simulink model "IPG"  (R2019a)
settings: Solver=FixedStepDiscrete  StartTime=0.0  StopTime=86.24  FixedStep=0.01  RelTol=1e-3
undefined symbols (not defined in the file): C1Prime, C2Prime, C3Prime, CapacityAh, DiscIntNeverNeededParam, Em, InitialCapVoltage, R0, Rx, SOC_LUT
settings Model: Creator=danis  LastModifiedBy=danis

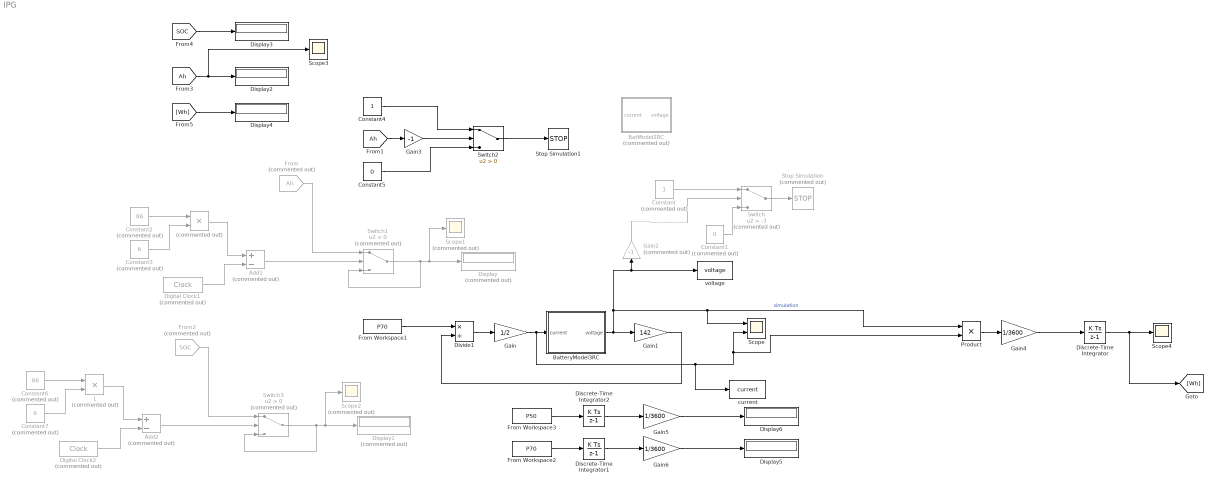
== system IPG ==
  " " : Product  Commented=on  Inputs=**
  " 1" : Product  Commented=on  Inputs=**
  Add1 : Sum  Commented=on  Inputs=+-
  Add2 : Sum  Commented=on  Inputs=+-
  BatModel2RC : Subsystem  Commented=on
  BatteryModel3RC : Subsystem
  Constant : Constant  Commented=on  SampleTime=0.01
  Constant1 : Constant  Commented=on  Value=0  SampleTime=0.01
  Constant2 : Constant  Commented=on  Value=86  SampleTime=0.01
  Constant3 : Constant  Commented=on  Value=6  SampleTime=0.01
  Constant4 : Constant  SampleTime=0.01
  Constant5 : Constant  Value=0  SampleTime=0.01
  Constant6 : Constant  Commented=on  Value=86  SampleTime=0.01
  Constant7 : Constant  Commented=on  Value=6  SampleTime=0.01
  Digital Clock1 : DigitalClock  Commented=on  SampleTime=0.01
  Digital Clock2 : DigitalClock  Commented=on  SampleTime=0.01
  Discrete-Time Integrator : DiscreteIntegrator  SampleTime=-1  ICPrevOutput=DiscIntNeverNeededParam  ICPrevScaledInput=DiscIntNeverNeededParam
  Discrete-Time Integrator1 : DiscreteIntegrator  SampleTime=-1  ICPrevOutput=DiscIntNeverNeededParam  ICPrevScaledInput=DiscIntNeverNeededParam
  Discrete-Time Integrator2 : DiscreteIntegrator  SampleTime=-1  ICPrevOutput=DiscIntNeverNeededParam  ICPrevScaledInput=DiscIntNeverNeededParam
  Display : Display  Commented=on
  Display1 : Display  Commented=on
  Display{2..6} (5 alike) : Display
  Divide1 : Product  Inputs=*/
  From : From  Commented=on  GotoTag=Ah  TagVisibility=global
  From Workspace1 : FromWorkspace  VariableName=P70  SampleTime=0.01  Interpolate=off  OutputAfterFinalValue=Cyclic repetition
  From Workspace2 : FromWorkspace  VariableName=P70  SampleTime=0.01  Interpolate=off  OutputAfterFinalValue=Cyclic repetition
  From Workspace3 : FromWorkspace  VariableName=P50  SampleTime=0.01  Interpolate=off  OutputAfterFinalValue=Cyclic repetition
  From2 : From  Commented=on  GotoTag=SOC  TagVisibility=global
  Gain : Gain  Gain=1/2
  Gain1 : Gain  Gain=142
  Gain2 : Gain  Commented=on  Gain=-1
  Gain3 : Gain  Gain=-1
  Gain4 : Gain  Gain=1/3600
  Gain5 : Gain  Gain=1/3600
  Gain6 : Gain  Gain=1/3600
  Product : Product
  Scope : Scope  NumInputPorts=2
  Scope1 : Scope  Commented=on
  Scope2 : Scope  Commented=on
  Scope3 : Scope
  Scope4 : Scope
  Stop Simulation : Stop  Commented=on
  Stop Simulation1 : Stop
  Switch : Switch  Commented=on  Criteria=u2 > Threshold  Threshold=-3
  Switch1 : Switch  Commented=on  Criteria=u2 > Threshold
  Switch2 : Switch  Criteria=u2 > Threshold
  Switch3 : Switch  Commented=on  Criteria=u2 > Threshold
  current : ToWorkspace  VariableName=current  SaveFormat=Structure With Time  SampleTime=-1
  voltage : ToWorkspace  VariableName=voltage  SaveFormat=Structure With Time  SampleTime=-1
  wires:
  Divide1/1 -> Gain/1
  Gain/1 -> BatteryModel3RC/1(current), current/1, Scope/2, Product/2
  Gain1/1 -> Divide1/2
  Switch/1 -> Stop Simulation/1
  Gain2/1 -> Switch/2
  Constant/1 -> Switch/1
  Constant1/1 -> Switch/3
  From Workspace1/1 -> Divide1/1
  From/1 -> Switch1/1
  Add1/1 -> Switch1/2
  Switch1/1 -> Switch1/3, Scope1/1, Display/1
  Constant2/1 -> " "/1
  Constant3/1 -> " "/2
  " "/1 -> Add1/1
  Digital Clock1/1 -> Add1/2
  [Ah] -> Gain3/1
  Constant4/1 -> Switch2/1
  Constant5/1 -> Switch2/3
  Switch2/1 -> Stop Simulation1/1
  Digital Clock2/1 -> Add2/2
  " 1"/1 -> Add2/1
  Constant7/1 -> " 1"/2
  Constant6/1 -> " 1"/1
  Switch3/1 -> Display1/1, Scope2/1, Switch3/3
  Add2/1 -> Switch3/2
  From2/1 -> Switch3/1
  Gain3/1 -> Switch2/2
  [Ah] -> Scope3/1, Display2/1
  [SOC] -> Display3/1
  Discrete-Time Integrator/1 -> [Wh], Scope4/1
  Gain4/1 -> Discrete-Time Integrator/1
  Product/1 -> Gain4/1
  [Wh] -> Display4/1
  BatteryModel3RC/1(voltage) -> Gain1/1, Product/1, Scope/1, voltage/1, Gain2/1  "simulation"
  From Workspace2/1 -> Discrete-Time Integrator1/1
  Discrete-Time Integrator1/1 -> Gain6/1
  Gain6/1 -> Display5/1
  Gain5/1 -> Display6/1
  Discrete-Time Integrator2/1 -> Gain5/1
  From Workspace3/1 -> Discrete-Time Integrator2/1

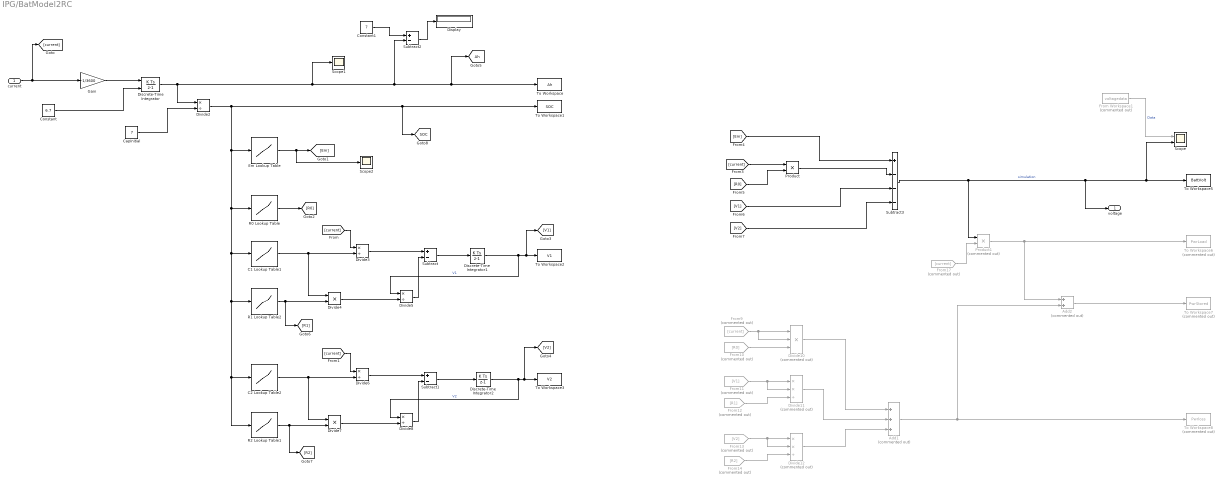
== system IPG/BatModel2RC ==
  current : Inport
  Add1 : Sum  Commented=on  Inputs=+++
  Add2 : Sum  Commented=on
  C1 Lookup Table1 : Lookup_n-D  NumberOfTableDimensions=1  BreakpointsForDimension1=SOC_LUT  Table=C1Prime(1,:)  InternalRulePriority=Speed  RndMeth=Simplest  InputSameDT=on
  C2 Lookup Table2 : Lookup_n-D  NumberOfTableDimensions=1  BreakpointsForDimension1=SOC_LUT  Table=C2Prime(1,:)  InternalRulePriority=Speed  RndMeth=Simplest  InputSameDT=on
  CapInitial : Constant  Value=7  SampleTime=-1
  Constant : Constant  Value=6.7  SampleTime=-1
  Constant1 : Constant  Value=7  SampleTime=0.01
  Discrete-Time Integrator : DiscreteIntegrator  InitialConditionSource=external  SampleTime=-1  ICPrevOutput=DiscIntNeverNeededParam  ICPrevScaledInput=DiscIntNeverNeededParam
  Discrete-Time Integrator1 : DiscreteIntegrator  InitialCondition=InitialCapVoltage(1)  SampleTime=-1  ICPrevOutput=DiscIntNeverNeededParam  ICPrevScaledInput=DiscIntNeverNeededParam
  Discrete-Time Integrator2 : DiscreteIntegrator  InitialCondition=InitialCapVoltage(2)  SampleTime=-1  ICPrevOutput=DiscIntNeverNeededParam  ICPrevScaledInput=DiscIntNeverNeededParam
  Display : Display
  Divide10 : Product  Commented=on  Inputs=***
  Divide11 : Product  Commented=on  Inputs=**/
  Divide12 : Product  Commented=on  Inputs=**/
  Divide{2..3,5..6,8} (5 alike) : Product  Inputs=*/
  Divide4 : Product  Inputs=**
  Divide7 : Product  Inputs=**
  Em Lookup Table : Lookup_n-D  NumberOfTableDimensions=1  BreakpointsForDimension1=SOC_LUT  Table=Em  InternalRulePriority=Speed  RndMeth=Simplest  InputSameDT=on
  From Workspace1 : FromWorkspace  Commented=on  VariableName=voltagedata  SampleTime=0.001
  From10 : From  Commented=on  GotoTag=R0
  From11 : From  Commented=on  GotoTag=V1
  From12 : From  Commented=on  GotoTag=R1
  From13 : From  Commented=on  GotoTag=V2
  From14 : From  Commented=on  GotoTag=R2
  From17 : From  Commented=on  GotoTag=current
  From9 : From  Commented=on  GotoTag=current
  Gain : Gain  Gain=-1/3600
  Product : Product
  Product1 : Product  Commented=on
  R0 Lookup Table : Lookup_n-D  NumberOfTableDimensions=1  BreakpointsForDimension1=SOC_LUT  Table=R0  InternalRulePriority=Speed  RndMeth=Simplest  InputSameDT=on
  R1 Lookup Table2 : Lookup_n-D  NumberOfTableDimensions=1  BreakpointsForDimension1=SOC_LUT  Table=Rx(1,:)  InternalRulePriority=Speed  RndMeth=Simplest  InputSameDT=on
  R2 Lookup Table1 : Lookup_n-D  NumberOfTableDimensions=1  BreakpointsForDimension1=SOC_LUT  Table=Rx(2,:)  InternalRulePriority=Speed  RndMeth=Simplest  InputSameDT=on
  Scope : Scope  NumInputPorts=2
  Scope1 : Scope
  Scope2 : Scope
  Subtract : Sum  Inputs=+-
  Subtract1 : Sum  Inputs=+-
  Subtract2 : Sum  Inputs=+-
  Subtract3 : Sum  Inputs=+---
  To Workspace : ToWorkspace  VariableName=Ah  SampleTime=-1
  To Workspace1 : ToWorkspace  VariableName=SOC  SampleTime=-1
  To Workspace2 : ToWorkspace  VariableName=V1  SampleTime=-1
  To Workspace3 : ToWorkspace  VariableName=V2  SampleTime=-1
  To Workspace5 : ToWorkspace  VariableName=BattVolt  SampleTime=-1
  To Workspace6 : ToWorkspace  Commented=on  VariableName=PwrLoad  SampleTime=-1
  To Workspace7 : ToWorkspace  Commented=on  VariableName=PwrStored  SampleTime=-1
  To Workspace8 : ToWorkspace  Commented=on  VariableName=Pwrloss  SampleTime=-1
  voltage : Outport
  tag scope: Ah=global, SOC=global
  wires:
  Gain/1 -> Discrete-Time Integrator/1
  Discrete-Time Integrator/1 -> Scope1/1, Subtract2/2, [Ah], To Workspace/1, Divide2/1
  Divide10/1 -> Add1/1
  Discrete-Time Integrator1/1 -> Divide5/1, To Workspace2/1, [V1]  "V1"
  Divide2/1 -> [SOC], To Workspace1/1, R2 Lookup Table1/1, C2 Lookup Table2/1, R1 Lookup Table2/1, C1 Lookup Table1/1, R0 Lookup Table/1, Em Lookup Table/1
  From12/1 -> Divide11/3
  Subtract3/1 -> voltage/1, To Workspace5/1, Scope/2, Product1/1  "simulation"
  From Workspace1/1 -> Scope/1  "Data"
  Divide11/1 -> Add1/2
  Divide8/1 -> Subtract1/2
  Add1/1 -> To Workspace8/1, Add2/2
  [Em] -> Subtract3/1
  Divide3/1 -> Subtract/1
  current/1 -> [current], Gain/1
  Discrete-Time Integrator2/1 -> Divide8/1, To Workspace3/1, [V2]  "V2"
  From9/1 -> Divide10/2, Divide10/1
  From11/1 -> Divide11/2, Divide11/1
  [current] -> Divide6/1
  Divide4/1 -> Divide5/2
  C1 Lookup Table1/1 -> Divide4/1, Divide3/2
  [V2] -> Subtract3/4
  Subtract/1 -> Discrete-Time Integrator1/1
  R1 Lookup Table2/1 -> [R1], Divide4/2
  Divide7/1 -> Divide8/2
  [R0] -> Product/2
  From13/1 -> Divide12/2, Divide12/1
  From17/1 -> Product1/2
  Subtract1/1 -> Discrete-Time Integrator2/1
  R2 Lookup Table1/1 -> [R2], Divide7/2
  R0 Lookup Table/1 -> [R0]
  CapInitial/1 -> Divide2/2
  Divide12/1 -> Add1/3
  Product1/1 -> To Workspace6/1, Add2/1
  Add2/1 -> To Workspace7/1
  [current] -> Divide3/1
  [current] -> Product/1
  C2 Lookup Table2/1 -> Divide7/1, Divide6/2
  [V1] -> Subtract3/3
  Divide6/1 -> Subtract1/1
  From14/1 -> Divide12/3
  From10/1 -> Divide10/3
  Product/1 -> Subtract3/2
  Divide5/1 -> Subtract/2
  Constant/1 -> Discrete-Time Integrator/2
  Em Lookup Table/1 -> Scope2/1, [Em]
  Constant1/1 -> Subtract2/1
  Subtract2/1 -> Display/1

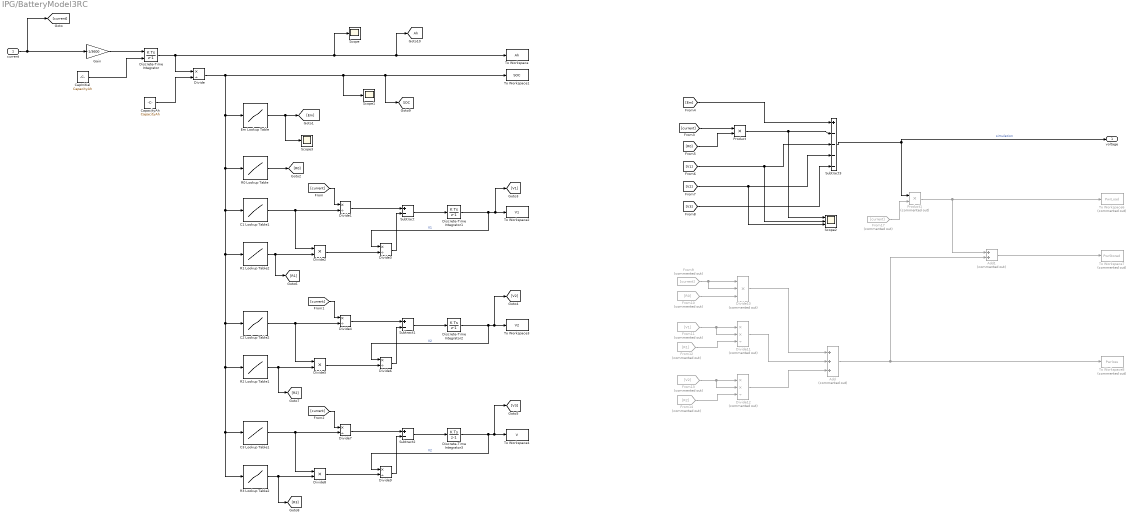
== system IPG/BatteryModel3RC ==
  current : Inport
  Add : Sum  Commented=on  Inputs=+++
  Add1 : Sum  Commented=on
  C1 Lookup Table1 : Lookup_n-D  NumberOfTableDimensions=1  BreakpointsForDimension1=SOC_LUT  Table=C1Prime(1,:)  InternalRulePriority=Speed  RndMeth=Simplest  InputSameDT=on
  C2 Lookup Table2 : Lookup_n-D  NumberOfTableDimensions=1  BreakpointsForDimension1=SOC_LUT  Table=C2Prime(1,:)  InternalRulePriority=Speed  RndMeth=Simplest  InputSameDT=on
  C3 Lookup Table1 : Lookup_n-D  NumberOfTableDimensions=1  BreakpointsForDimension1=SOC_LUT  Table=C3Prime(1,:)  InternalRulePriority=Speed  RndMeth=Simplest  InputSameDT=on
  CapInitial : Constant  Value=CapacityAh  SampleTime=-1
  CapacityAh : Constant  Value=CapacityAh  SampleTime=-1
  Discrete-Time Integrator : DiscreteIntegrator  InitialConditionSource=external  SampleTime=-1  ICPrevOutput=DiscIntNeverNeededParam  ICPrevScaledInput=DiscIntNeverNeededParam
  Discrete-Time Integrator1 : DiscreteIntegrator  SampleTime=-1  ICPrevOutput=DiscIntNeverNeededParam  ICPrevScaledInput=DiscIntNeverNeededParam
  Discrete-Time Integrator2 : DiscreteIntegrator  SampleTime=-1  ICPrevOutput=DiscIntNeverNeededParam  ICPrevScaledInput=DiscIntNeverNeededParam
  Discrete-Time Integrator3 : DiscreteIntegrator  SampleTime=-1  ICPrevOutput=DiscIntNeverNeededParam  ICPrevScaledInput=DiscIntNeverNeededParam
  Divide{,1,3..4,6..7,9} (7 alike) : Product  Inputs=*/
  Divide10 : Product  Commented=on  Inputs=***
  Divide11 : Product  Commented=on  Inputs=**/
  Divide12 : Product  Commented=on  Inputs=**/
  Divide2 : Product  Inputs=**
  Divide5 : Product  Inputs=**
  Divide8 : Product  Inputs=**
  Em Lookup Table : Lookup_n-D  NumberOfTableDimensions=1  BreakpointsForDimension1=SOC_LUT  Table=Em  InternalRulePriority=Speed  RndMeth=Simplest  InputSameDT=on
  From10 : From  Commented=on  GotoTag=R0
  From11 : From  Commented=on  GotoTag=V1
  From12 : From  Commented=on  GotoTag=R1
  From13 : From  Commented=on  GotoTag=V2
  From14 : From  Commented=on  GotoTag=R2
  From17 : From  Commented=on  GotoTag=current
  From9 : From  Commented=on  GotoTag=current
  Gain : Gain  Gain=-1/3600
  Product : Product
  Product1 : Product  Commented=on
  R0 Lookup Table : Lookup_n-D  NumberOfTableDimensions=1  BreakpointsForDimension1=SOC_LUT  Table=R0  InternalRulePriority=Speed  RndMeth=Simplest  InputSameDT=on
  R1 Lookup Table2 : Lookup_n-D  NumberOfTableDimensions=1  BreakpointsForDimension1=SOC_LUT  Table=Rx(1,:)  InternalRulePriority=Speed  RndMeth=Simplest  InputSameDT=on
  R2 Lookup Table1 : Lookup_n-D  NumberOfTableDimensions=1  BreakpointsForDimension1=SOC_LUT  Table=Rx(2,:)  InternalRulePriority=Speed  RndMeth=Simplest  InputSameDT=on
  R3 Lookup Table2 : Lookup_n-D  NumberOfTableDimensions=1  BreakpointsForDimension1=SOC_LUT  Table=Rx(3,:)  InternalRulePriority=Speed  RndMeth=Simplest  InputSameDT=on
  Scope : Scope
  Scope1 : Scope
  Scope2 : Scope  NumInputPorts=3
  Scope3 : Scope
  Subtract : Sum  Inputs=+-
  Subtract1 : Sum  Inputs=+-
  Subtract2 : Sum  Inputs=+-
  Subtract3 : Sum  Inputs=+----
  To Workspace : ToWorkspace  VariableName=Ah  SampleTime=-1
  To Workspace1 : ToWorkspace  VariableName=SOC  SampleTime=-1
  To Workspace2 : ToWorkspace  VariableName=V1  SampleTime=-1
  To Workspace3 : ToWorkspace  VariableName=V2  SampleTime=-1
  To Workspace4 : ToWorkspace  VariableName=V  SampleTime=-1
  To Workspace6 : ToWorkspace  Commented=on  VariableName=PwrLoad  SampleTime=-1
  To Workspace7 : ToWorkspace  Commented=on  VariableName=PwrStored  SampleTime=-1
  To Workspace8 : ToWorkspace  Commented=on  VariableName=Pwrloss  SampleTime=-1
  voltage : Outport
  tag scope: Ah=global, SOC=global
  wires:
  Discrete-Time Integrator2/1 -> Divide6/1, To Workspace3/1, [V2]  "V2"
  Divide4/1 -> Subtract1/1
  [R0] -> Product/2
  Discrete-Time Integrator/1 -> Scope/1, [Ah], To Workspace/1, Divide/1
  C2 Lookup Table2/1 -> Divide5/1, Divide4/2
  C1 Lookup Table1/1 -> Divide2/1, Divide1/2
  Gain/1 -> Discrete-Time Integrator/1
  From17/1 -> Product1/2
  Divide3/1 -> Subtract/2
  Divide6/1 -> Subtract1/2
  [Em] -> Subtract3/1
  Divide5/1 -> Divide6/2
  Subtract/1 -> Discrete-Time Integrator1/1
  R2 Lookup Table1/1 -> [R2], Divide5/2
  Divide2/1 -> Divide3/2
  Divide1/1 -> Subtract/1
  CapacityAh/1 -> Divide/2
  From9/1 -> Divide10/2, Divide10/1
  Discrete-Time Integrator1/1 -> Divide3/1, To Workspace2/1, [V1]  "V1"
  Divide10/1 -> Add/1
  From11/1 -> Divide11/2, Divide11/1
  Subtract1/1 -> Discrete-Time Integrator2/1
  [current] -> Product/1
  [current] -> Divide4/1
  [V2] -> Scope2/3, Subtract3/4
  From12/1 -> Divide11/3
  R1 Lookup Table2/1 -> [R1], Divide2/2
  Product/1 -> Scope2/1, Subtract3/2
  Em Lookup Table/1 -> Scope3/1, [Em]
  [V1] -> Scope2/2, Subtract3/3
  From10/1 -> Divide10/3
  Divide11/1 -> Add/2
  [current] -> Divide1/1
  Divide12/1 -> Add/3
  R0 Lookup Table/1 -> [R0]
  From14/1 -> Divide12/3
  Subtract3/1 -> voltage/1, Product1/1  "simulation"
  Add1/1 -> To Workspace7/1
  From13/1 -> Divide12/2, Divide12/1
  Add/1 -> To Workspace8/1, Add1/2
  Product1/1 -> To Workspace6/1, Add1/1
  current/1 -> [current], Gain/1
  CapInitial/1 -> Discrete-Time Integrator/2
  [current] -> Divide7/1
  Subtract2/1 -> Discrete-Time Integrator3/1
  Divide/1 -> Scope1/1, [SOC], To Workspace1/1, C3 Lookup Table1/1, R3 Lookup Table2/1, R2 Lookup Table1/1, C2 Lookup Table2/1, R1 Lookup Table2/1, C1 Lookup Table1/1, R0 Lookup Table/1, Em Lookup Table/1
  R3 Lookup Table2/1 -> Divide8/2, [R3]
  Divide8/1 -> Divide9/2
  Divide9/1 -> Subtract2/2
  C3 Lookup Table1/1 -> Divide7/2, Divide8/1
  Divide7/1 -> Subtract2/1
  Discrete-Time Integrator3/1 -> [V3], To Workspace4/1, Divide9/1  "V2"
  [V3] -> Subtract3/5
